simulink model "lista1_questao3"  (R2014b)
settings: Solver=ode45  StartTime=0.0  StopTime=20  RelTol=1e-3
settings Model: Creator=Danilo  LastModifiedBy=Danilo

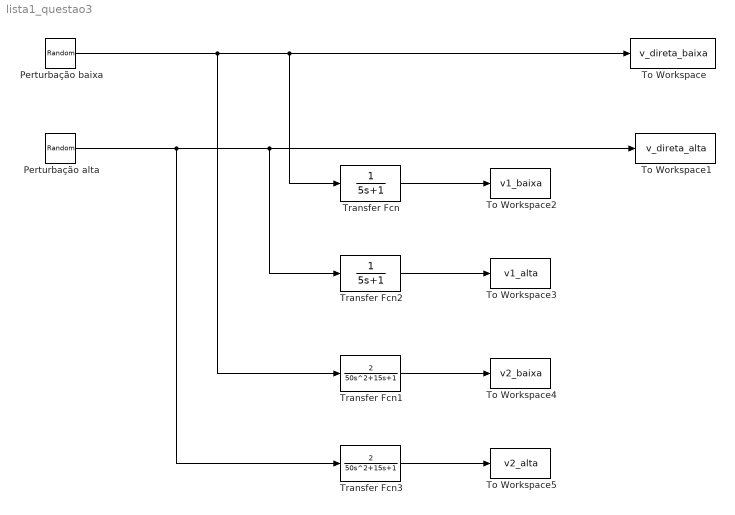
== system lista1_questao3 ==
  "Perturbação alta " : RandomNumber  Variance=0.1  SampleTime=0.1
  Perturbação baixa : RandomNumber  Variance=0.001  SampleTime=0.1
  To Workspace : ToWorkspace  VariableName=v_direta_baixa  SaveFormat=Timeseries  SampleTime=-1
  To Workspace1 : ToWorkspace  VariableName=v_direta_alta  SaveFormat=Timeseries  SampleTime=-1
  To Workspace2 : ToWorkspace  VariableName=v1_baixa  SaveFormat=Timeseries  SampleTime=-1
  To Workspace3 : ToWorkspace  VariableName=v1_alta  SaveFormat=Timeseries  SampleTime=-1
  To Workspace4 : ToWorkspace  VariableName=v2_baixa  SaveFormat=Timeseries  SampleTime=-1
  To Workspace5 : ToWorkspace  VariableName=v2_alta  SaveFormat=Timeseries  SampleTime=-1
  Transfer Fcn : TransferFcn  Denominator=[5 1]
  Transfer Fcn1 : TransferFcn  Numerator=[2]  Denominator=[50 15 1]
  Transfer Fcn2 : TransferFcn  Denominator=[5 1]
  Transfer Fcn3 : TransferFcn  Numerator=[2]  Denominator=[50 15 1]
  wires:
  "Perturbação alta "/1 -> Transfer Fcn3/1, Transfer Fcn2/1, To Workspace1/1
  Transfer Fcn/1 -> To Workspace2/1
  Transfer Fcn1/1 -> To Workspace4/1
  Transfer Fcn2/1 -> To Workspace3/1
  Transfer Fcn3/1 -> To Workspace5/1
  Perturbação baixa/1 -> Transfer Fcn1/1, Transfer Fcn/1, To Workspace/1
